simulink model "Open_Loop_Gust_Response"  (R2023a)
settings: Solver=FixedStepDiscrete  StartTime=0.0  StopTime=input_settings.flight_time  FixedStep=input_settings.dt  RelTol=1e-3
undefined symbols (not defined in the file): control_surface_mapping, input_settings, linear_sys
settings Model: Creator=sjd320  LastModifiedBy=sduess
settings DebuggingCC: UnconnectedInputMsg=warning  UnconnectedOutputMsg=warning  UnconnectedLineMsg=warning
settings ModelReferenceCC: EnableRefExpFcnMdlSchedulingChecks=on
settings RTWCC: DLArmComputeVersion=19.05

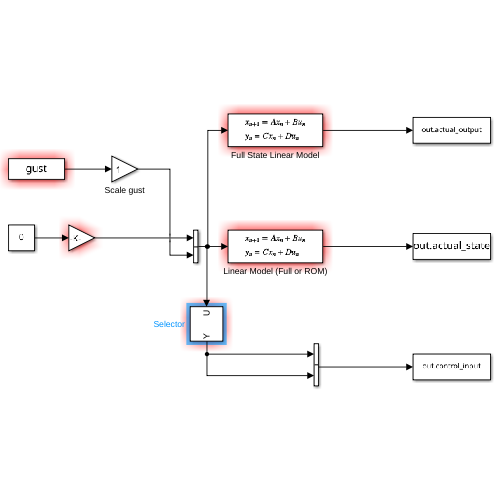
[thumbnail: Simulink's stored preview of the top-level diagram]
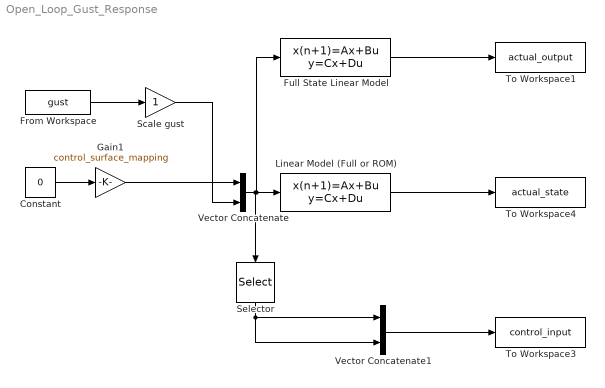
== system Open_Loop_Gust_Response ==
  Constant : Constant  Value=0
  From Workspace : FromWorkspace  VariableName=gust  SampleTime=-1
  Full State Linear Model : DiscreteStateSpace  A=linear_sys.A  B=linear_sys.B  C=linear_sys.C  D=linear_sys.D  SampleTime=input_settings.dt
  Gain1 : Gain  Gain=control_surface_mapping
  Linear Model (Full or ROM) : DiscreteStateSpace  A=linear_sys.A  B=linear_sys.B  C=eye(size(linear_sys.A,1))  D=linear_sys.B .* 0.  SampleTime=input_settings.dt
  Scale gust : Gain
  Selector : Selector  InputPortWidth=size(linear_sys.B,2)  IndexOptions=Index vector (dialog)  Indices=1:size(linear_sys.B,2)-1  OutputSizes=1
  To Workspace1 : ToWorkspace  VariableName=actual_output  SaveFormat=Timeseries  SampleTime=-1
  To Workspace3 : ToWorkspace  VariableName=control_input  SaveFormat=Timeseries  SampleTime=-1
  To Workspace4 : ToWorkspace  VariableName=actual_state  SaveFormat=Timeseries  SampleTime=-1
  Vector Concatenate : Concatenate
  Vector Concatenate1 : Concatenate
  wires:
  Vector Concatenate/1 -> Full State Linear Model/1, Linear Model (Full or ROM)/1, Selector/1
  From Workspace/1 -> Scale gust/1
  Scale gust/1 -> Vector Concatenate/2
  Full State Linear Model/1 -> To Workspace1/1
  Linear Model (Full or ROM)/1 -> To Workspace4/1
  Vector Concatenate1/1 -> To Workspace3/1
  Constant/1 -> Gain1/1
  Gain1/1 -> Vector Concatenate/1
  Selector/1 -> Vector Concatenate1/2, Vector Concatenate1/1
